simulink library "qss_tb_library"  (Simulink 10.0)
settings: Solver=ode45  StartTime=0.0  StopTime=1220  RelTol=1e-3
undefined symbols (not defined in the file): automatic_gearbox, cc_done, delta_h_C_air, DiscIntNeverNeededParam, dw_GG_c, eta_EG_map, eta_EM_map, eta_ice, g, h, H_o_m, H_u, i_FC_in, i_FC_max, k1, k2, k3, k4, k_cs, M_air, manual_gearbox, P_aux, P_CE_cutoff, P_CE_idle, P_CE_recup, P_CVT_opt, Q_BT_min, Q_SC_IC, r, rho, rho_f, t_c, T_CE_cutoff, T_CE_max, T_EG_c, T_EG_max, T_EM_max, theta_CE, theta_EM, V_CE_map, V_FC_out, w_CE_idle, w_CE_max, w_CE_upper, w_CVT_opt, w_EG_row, w_EG_upper, w_EM_row, w_EM_upper, w_GG_c
(part 4 of 4)

== system qss_tb_library/Gear System/Manual Gear Box/Power flow/Engine -> Wheel ==
  w_wheel : Inport
  T_wheel : Inport  Port=2
  gear : Inport  Port=3
  Constant1 : Constant  Value=P_GT0
  Constant2 : Constant  Value=inf
  Gain : Gain  Gain=e_GT  SaturateOnIntegerOverflow=on  OutDataTypeStr=Inherit: Same as input  ParamDataTypeStr=Inherit: Same as input
  Product2 : Product  Inputs=*/  SaturateOnIntegerOverflow=on  RndMeth=Zero  InputSameDT=on  OutDataTypeStr=Inherit: Same as first input
  Product3 : Product  Inputs=/*  SaturateOnIntegerOverflow=on  RndMeth=Zero  InputSameDT=on  OutDataTypeStr=Inherit: Same as first input
  Sum : Sum  SaturateOnIntegerOverflow=on  InputSameDT=on  OutDataTypeStr=Inherit: Same as first input
  Switch1 : Switch  Threshold=w_wheel_min  SaturateOnIntegerOverflow=on  InputSameDT=on
  T_MGB+ : Outport  InitialOutput=0
  wires:
  T_wheel/1 -> Sum/2
  Product3/1 -> Sum/1
  Gain/1 -> Product2/2
  Product2/1 -> T_MGB+/1
  Sum/1 -> Product2/1
  w_wheel/1 -> Switch1/2, Switch1/1
  Constant2/1 -> Switch1/3
  Switch1/1 -> Product3/1
  Constant1/1 -> Product3/2
  gear/1 -> Gain/1

== system qss_tb_library/Gear System/Manual Gear Box/Power flow/Wheel -> Engine ==
  w_wheel : Inport
  T_wheel : Inport  Port=2
  gear : Inport  Port=3
  Constant1 : Constant  Value=P_GT0
  Constant2 : Constant  Value=inf
  Gain1 : Gain  Gain=e_GT  SaturateOnIntegerOverflow=on  OutDataTypeStr=Inherit: Same as input  ParamDataTypeStr=Inherit: Same as input
  Gain2 : Gain  Gain=1/e_GT  SaturateOnIntegerOverflow=on  OutDataTypeStr=Inherit: Same as input  ParamDataTypeStr=Inherit: Same as input
  Product2 : Product  Inputs=*/  SaturateOnIntegerOverflow=on  RndMeth=Zero  InputSameDT=on  OutDataTypeStr=Inherit: Same as first input
  Product3 : Product  Inputs=/*  SaturateOnIntegerOverflow=on  RndMeth=Zero  InputSameDT=on  OutDataTypeStr=Inherit: Same as first input
  Sum : Sum  SaturateOnIntegerOverflow=on  InputSameDT=on  OutDataTypeStr=Inherit: Same as first input
  Switch1 : Switch  Threshold=w_wheel_min  SaturateOnIntegerOverflow=on  InputSameDT=on
  T_MGB- : Outport  InitialOutput=0
  wires:
  w_wheel/1 -> Switch1/1, Switch1/2
  gear/1 -> Gain2/1
  Constant2/1 -> Switch1/3
  Switch1/1 -> Gain1/1
  Constant1/1 -> Product3/2
  T_wheel/1 -> Sum/1
  Gain2/1 -> Product2/2
  Product2/1 -> T_MGB-/1
  Product3/1 -> Sum/2
  Sum/1 -> Product2/1
  Gain1/1 -> Product3/1

== system qss_tb_library/Gear System/Simple Transmission/Power flow/Energy Engine -> Wheel ==
  w_wheel : Inport
  T_wheel : Inport  Port=2
  gear_ratio : Inport  Port=3
  Constant1 : Constant  Value=P_GT0
  Constant2 : Constant  Value=inf
  Gain : Gain  Gain=e_GT  SaturateOnIntegerOverflow=on  OutDataTypeStr=Inherit: Same as input  ParamDataTypeStr=Inherit: Same as input
  Product2 : Product  Inputs=*/  SaturateOnIntegerOverflow=on  RndMeth=Zero  InputSameDT=on  OutDataTypeStr=Inherit: Same as first input
  Product3 : Product  Inputs=/*  SaturateOnIntegerOverflow=on  RndMeth=Zero  InputSameDT=on  OutDataTypeStr=Inherit: Same as first input
  Sum : Sum  SaturateOnIntegerOverflow=on  InputSameDT=on  OutDataTypeStr=Inherit: Same as first input
  Switch1 : Switch  Threshold=w_wheel_min  SaturateOnIntegerOverflow=on  InputSameDT=on
  T_trans+ : Outport  InitialOutput=0
  wires:
  gear_ratio/1 -> Gain/1
  Constant1/1 -> Product3/2
  Switch1/1 -> Product3/1
  Constant2/1 -> Switch1/3
  w_wheel/1 -> Switch1/1, Switch1/2
  Sum/1 -> Product2/1
  Product2/1 -> T_trans+/1
  Gain/1 -> Product2/2
  Product3/1 -> Sum/1
  T_wheel/1 -> Sum/2

== system qss_tb_library/Gear System/Simple Transmission/Power flow/Energy Wheel -> Engine ==
  w_wheel : Inport
  T_wheel : Inport  Port=2
  gear_ratio : Inport  Port=3
  Constant1 : Constant  Value=P_GT0
  Constant2 : Constant  Value=inf
  Gain1 : Gain  Gain=e_GT  SaturateOnIntegerOverflow=on  OutDataTypeStr=Inherit: Same as input  ParamDataTypeStr=Inherit: Same as input
  Gain2 : Gain  Gain=1/e_GT  SaturateOnIntegerOverflow=on  OutDataTypeStr=Inherit: Same as input  ParamDataTypeStr=Inherit: Same as input
  Product2 : Product  Inputs=*/  SaturateOnIntegerOverflow=on  RndMeth=Zero  InputSameDT=on  OutDataTypeStr=Inherit: Same as first input
  Product3 : Product  Inputs=/*  SaturateOnIntegerOverflow=on  RndMeth=Zero  InputSameDT=on  OutDataTypeStr=Inherit: Same as first input
  Sum : Sum  SaturateOnIntegerOverflow=on  InputSameDT=on  OutDataTypeStr=Inherit: Same as first input
  Switch1 : Switch  Threshold=w_wheel_min  SaturateOnIntegerOverflow=on  InputSameDT=on
  T_trans- : Outport  InitialOutput=0
  wires:
  Gain1/1 -> Product3/1
  Sum/1 -> Product2/1
  Product3/1 -> Sum/2
  Product2/1 -> T_trans-/1
  Gain2/1 -> Product2/2
  T_wheel/1 -> Sum/1
  Constant1/1 -> Product3/2
  Switch1/1 -> Gain1/1
  Constant2/1 -> Switch1/3
  gear_ratio/1 -> Gain2/1
  w_wheel/1 -> Switch1/2, Switch1/1

== matlab function Energy Buffer/PHEV Battery/Cell electrical model/Stop Function/MATLAB Function ==
  data: u input double; y output double
function y = fcn(u)
coder.extrinsic('sprintf')
coder.extrinsic('helpdlg')

if u == 1
helpdlg(sprintf('Battery Charge Current Too High'))
else
end
y = u;

== matlab function Energy Buffer/PHEV Battery/Cell electrical model/Stop Function/MATLAB Function1 ==
  data: u input double; y output double
function y = fcn(u)
coder.extrinsic('sprintf')
coder.extrinsic('helpdlg')

if u == 1
helpdlg(sprintf('High Battery Discharge Current'))
else
end
y = u;

== matlab function Energy Buffer/PHEV Battery/Cell electrical model/Stop Function/MATLAB Function2 ==
  data: u input double; y output double
function y = fcn(u)
coder.extrinsic('sprintf')
coder.extrinsic('helpdlg')

if u == 1
helpdlg(sprintf('Upper SOC Limit'))
else
end
y = u;

== matlab function Energy Buffer/PHEV Battery/Cell electrical model/Stop Function/MATLAB Function3 ==
  data: u input double; y output double
function y = fcn(u)
coder.extrinsic('sprintf')
coder.extrinsic('helpdlg')

if u == 1
helpdlg(sprintf('Lower SOC Limit'))
else
end
y = u;

== matlab function Energy Buffer/BEV Battery/Cell electrical model/Stop Function/MATLAB Function ==
  data: u input double; y output double
function y = fcn(u)
coder.extrinsic('sprintf')
coder.extrinsic('helpdlg')

if u == 1
helpdlg(sprintf('Battery Charge Current Too High'))
else
end
y = u;

== matlab function Energy Buffer/BEV Battery/Cell electrical model/Stop Function/MATLAB Function1 ==
  data: u input double; y output double
function y = fcn(u)
coder.extrinsic('sprintf')
coder.extrinsic('helpdlg')

if u == 1
helpdlg(sprintf('High Battery Discharge Current'))
else
end
y = u;

== matlab function Energy Buffer/BEV Battery/Cell electrical model/Stop Function/MATLAB Function2 ==
  data: u input double; y output double
function y = fcn(u)
coder.extrinsic('sprintf')
coder.extrinsic('helpdlg')

if u == 1
helpdlg(sprintf('Upper SOC Limit'))
else
end
y = u;

== matlab function Energy Buffer/BEV Battery/Cell electrical model/Stop Function/MATLAB Function3 ==
  data: u input double; y output double
function y = fcn(u)
coder.extrinsic('sprintf')
coder.extrinsic('helpdlg')

if u == 1
helpdlg(sprintf('Lower SOC Limit'))
else
end
y = u;

== matlab function Energy Buffer/BEV Battery/Cell electrical model/Stop Function/MATLAB Function4 ==
  data: u input double; y output double
function y = fcn(u)
coder.extrinsic('sprintf')
coder.extrinsic('helpdlg')

if u == 1
helpdlg(sprintf('Cell Voltage Too High'))
else
end
y = u;

== matlab function Energy Buffer/BEV Battery/Cell electrical model/Stop Function/MATLAB Function5 ==
  data: u input double; y output double
function y = fcn(u)
coder.extrinsic('sprintf')
coder.extrinsic('helpdlg')

if u == 1
helpdlg(sprintf('Low Cell Voltage'))
else
end
y = u;

== matlab function Energy Buffer/PHEV Battery/Cell electrical model/Stop Function/MATLAB Function4 ==
  data: u input double; y output double
function y = fcn(u)
coder.extrinsic('sprintf')
coder.extrinsic('helpdlg')

if u == 1
helpdlg(sprintf('Cell Voltage Too High'))
else
end
y = u;

== matlab function Energy Buffer/PHEV Battery/Cell electrical model/Stop Function/MATLAB Function5 ==
  data: u input double; y output double
function y = fcn(u)
coder.extrinsic('sprintf')
coder.extrinsic('helpdlg')

if u == 1
helpdlg(sprintf('Low Cell Voltage'))
else
end
y = u;

== matlab function Energy Buffer/HEV Battery/Cell electrical model/Stop Function/MATLAB Function ==
  data: u input double; y output double
function y = fcn(u)
coder.extrinsic('sprintf')
coder.extrinsic('helpdlg')

if u == 1
helpdlg(sprintf('Battery Charge Current Too High'))
else
end
y = u;

== matlab function Energy Buffer/HEV Battery/Cell electrical model/Stop Function/MATLAB Function1 ==
  data: u input double; y output double
function y = fcn(u)
coder.extrinsic('sprintf')
coder.extrinsic('helpdlg')

if u == 1
helpdlg(sprintf('High Battery Discharge Current'))
else
end
y = u;

== matlab function Energy Buffer/HEV Battery/Cell electrical model/Stop Function/MATLAB Function2 ==
  data: u input double; y output double
function y = fcn(u)
coder.extrinsic('sprintf')
coder.extrinsic('helpdlg')

if u == 1
helpdlg(sprintf('Upper SOC Limit'))
else
end
y = u;

== matlab function Energy Buffer/HEV Battery/Cell electrical model/Stop Function/MATLAB Function3 ==
  data: u input double; y output double
function y = fcn(u)
coder.extrinsic('sprintf')
coder.extrinsic('helpdlg')

if u == 1
helpdlg(sprintf('Lower SOC Limit'))
else
end
y = u;

== matlab function Energy Buffer/HEV Battery/Cell electrical model/Stop Function/MATLAB Function4 ==
  data: u input double; y output double
function y = fcn(u)
coder.extrinsic('sprintf')
coder.extrinsic('helpdlg')

if u == 1
helpdlg(sprintf('Cell Voltage Too High'))
else
end
y = u;

== matlab function Energy Buffer/HEV Battery/Cell electrical model/Stop Function/MATLAB Function5 ==
  data: u input double; y output double
function y = fcn(u)
coder.extrinsic('sprintf')
coder.extrinsic('helpdlg')

if u == 1
helpdlg(sprintf('Low Cell Voltage'))
else
end
y = u;

== matlab function Energy Buffer/48V Battery/Cell electrical model/Stop Function/MATLAB Function ==
  data: u input double; y output double
function y = fcn(u)
coder.extrinsic('sprintf')
coder.extrinsic('helpdlg')

if u == 1
helpdlg(sprintf('Battery Charge Current Too High'))
else
end
y = u;

== matlab function Energy Buffer/48V Battery/Cell electrical model/Stop Function/MATLAB Function1 ==
  data: u input double; y output double
function y = fcn(u)
coder.extrinsic('sprintf')
coder.extrinsic('helpdlg')

if u == 1
helpdlg(sprintf('High Battery Discharge Current'))
else
end
y = u;

== matlab function Energy Buffer/48V Battery/Cell electrical model/Stop Function/MATLAB Function2 ==
  data: u input double; y output double
function y = fcn(u)
coder.extrinsic('sprintf')
coder.extrinsic('helpdlg')

if u == 1
helpdlg(sprintf('Upper SOC Limit'))
else
end
y = u;

== matlab function Energy Buffer/48V Battery/Cell electrical model/Stop Function/MATLAB Function3 ==
  data: u input double; y output double
function y = fcn(u)
coder.extrinsic('sprintf')
coder.extrinsic('helpdlg')

if u == 1
helpdlg(sprintf('Lower SOC Limit'))
else
end
y = u;

== matlab function Energy Buffer/48V Battery/Cell electrical model/Stop Function/MATLAB Function4 ==
  data: u input double; y output double
function y = fcn(u)
coder.extrinsic('sprintf')
coder.extrinsic('helpdlg')

if u == 1
helpdlg(sprintf('Cell Voltage Too High'))
else
end
y = u;

== matlab function Energy Buffer/48V Battery/Cell electrical model/Stop Function/MATLAB Function5 ==
  data: u input double; y output double
function y = fcn(u)
coder.extrinsic('sprintf')
coder.extrinsic('helpdlg')

if u == 1
helpdlg(sprintf('Low Cell Voltage'))
else
end
y = u;

== matlab function Energy Buffer/Battery Assignment/Cell electrical model/Stop Function/MATLAB Function ==
  data: u input double; y output double
function y = fcn(u)
coder.extrinsic('sprintf')
coder.extrinsic('helpdlg')

if u == 1
helpdlg(sprintf('Battery Charge Current Too High'))
else
end
y = u;

== matlab function Energy Buffer/Battery Assignment/Cell electrical model/Stop Function/MATLAB Function1 ==
  data: u input double; y output double
function y = fcn(u)
coder.extrinsic('sprintf')
coder.extrinsic('helpdlg')

if u == 1
helpdlg(sprintf('High Battery Discharge Current'))
else
end
y = u;

== matlab function Energy Buffer/Battery Assignment/Cell electrical model/Stop Function/MATLAB Function2 ==
  data: u input double; y output double
function y = fcn(u)
coder.extrinsic('sprintf')
coder.extrinsic('helpdlg')

if u == 1
helpdlg(sprintf('Upper SOC Limit'))
else
end
y = u;

== matlab function Energy Buffer/Battery Assignment/Cell electrical model/Stop Function/MATLAB Function3 ==
  data: u input double; y output double
function y = fcn(u)
coder.extrinsic('sprintf')
coder.extrinsic('helpdlg')

if u == 1
helpdlg(sprintf('Lower SOC Limit'))
else
end
y = u;

== matlab function Energy Buffer/Battery Assignment/Cell electrical model/Stop Function/MATLAB Function4 ==
  data: u input double; y output double
function y = fcn(u)
coder.extrinsic('sprintf')
coder.extrinsic('helpdlg')

if u == 1
helpdlg(sprintf('Cell Voltage Too High'))
else
end
y = u;

== matlab function Energy Buffer/Battery Assignment/Cell electrical model/Stop Function/MATLAB Function5 ==
  data: u input double; y output double
function y = fcn(u)
coder.extrinsic('sprintf')
coder.extrinsic('helpdlg')

if u == 1
helpdlg(sprintf('Low Cell Voltage'))
else
end
y = u;
